simulink model "Automata_Codesys"  (R2018a)
settings: Solver=VariableStepAuto  StartTime=0.0  StopTime=inf  RelTol=1e-3
values from neighbouring files (symbols this model uses):
  bcx = 1000e3    (= 1000000)    [Variables.m]
  bcy = 500e3    (= 500000)    [Variables.m]
  beq1 = 30    [Variables.m]
  beq2 = 18    [Variables.m]
  bw = 30000    [Variables.m]
  g = 9.81    [Variables.m]
  Jeq1 = Jwc+Jmc*(rc^2)    (= 2252)    [Variables.m]
  Jeq2 = Jd+Jmi*(riz^2)    (= 27008)    [Variables.m]
  kcy = 1.3e11    (= 130000000000)    [Variables.m]
  Kw = 1800e3    (= 1800000)    [Variables.m]
  Mc = 50000    [Variables.m]
  Mt = Mc+Jeq1*(1/(Rw^2))    (= 59008)    [Variables.m]
  rc = 15    [Variables.m]
  Rd = 0.75    [Variables.m]
  riz = 30    [Variables.m]
  Rw = 0.5    [Variables.m]
  Y_t0 = 45    [Variables.m]
undefined symbols (not defined in the file or in its folder): AlturaInicialBarco, AlturaInicialMuelle, cont_muelle_masa, contenedores, PObjetivo_fijo, PObjetivo_incremental, x_der, x_izq, Y_inf_barco, Y_max, Y_muelle, Y_sb
libraries: opclib x5
settings Model: Creator=Santiago  LastModifiedBy=Santiago

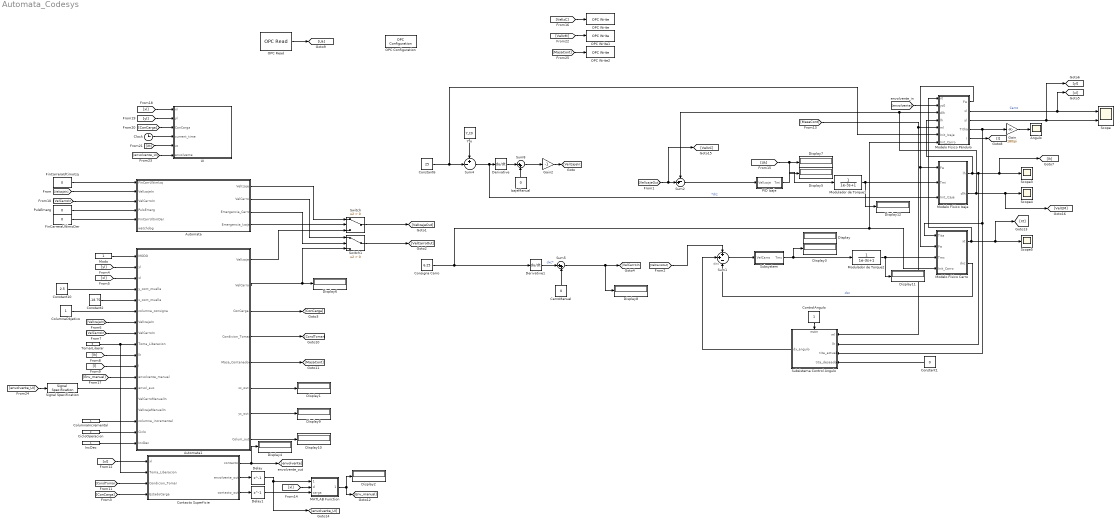
== system Automata_Codesys ==
  note: dxc
  Angulo : Scope
  Automata : Stateflow chart  TreatAsAtomicUnit=on
  Automata1 : Stateflow chart  TreatAsAtomicUnit=on
  CarroManual : Constant  Value=0
  CicloOperacion : Constant  Value=2
  Clock : Clock
  ColumnaIncremental : Constant
  ColumnaObjetivo : Constant
  Consigna Carro : Constant  Value=6.25
  Constant1 : Constant  Value=0
  Constant10 : Constant  Value=2.5
  Constant2 : Constant  Value=-18.75
  Constant6 : Constant  Value=25
  Contacto Superficie : Stateflow chart  TreatAsAtomicUnit=on
  ControlAngulo : Constant
  Delay : Delay  DelayLength=1  InitialCondition=0
  Delay1 : Delay  DelayLength=1  InitialCondition=0
  Derivative : Derivative
  Derivative1 : Derivative
  Display{,1..12} (13 alike) : Display
  FinCarreraUltimoDer : Constant  Value=0
  FinCarreraUltimoIzq : Constant  Value=0
  Gain : Gain  Gain=180/pi
  Gain2 : Gain  Gain=-1
  IncDec : Constant
  IzajeManual : Constant  Value=0
  MATLAB Function : MATLAB Function  TreatAsAtomicUnit=on
  "Modelo Físico Carro " : Subsystem
  Modelo Físico Izaje : Subsystem
  "Modelo Físico Péndulo " : Subsystem
  Modo : Constant
  Modulador de Torque1 : TransferFcn  Denominator=[1e-3 1]
  Modulador de Torque2 : TransferFcn  Denominator=[1e-3 1]
  OPC Configuration : opclib/OPC Configuration  opcServers=localhost/CoDeSys.OPC.DA/100  errMissingItems=Error  errReadWrite=Warn  errShutdown=Error  errRTViolation=Warn  rtEnable=on  speedup=1  showLatency=off  beingUsed=on
      settings: SourceProductName=OPC Toolbox  SourceProductBaseCode=OT
  OPC Read : opclib/OPC Read  serverHost=localhost  serverID=CoDeSys.OPC.DA  itemIDs=Automata.Application.SFC_NIVEL_2.Uk  readMode=Synchronous (cache)  dataType=double  updateRate=1  showQual=off  showTS=off  tsMode=Seconds since start
      settings: SourceProductName=OPC Toolbox  SourceProductBaseCode=OT
  OPC Write : opclib/OPC Write  serverHost=localhost  serverID=CoDeSys.OPC.DA  itemIDs=Automata.Application.SFC_NIVEL_2.VelIzc  writeMode=Synchronous  updateRate=1
      settings: SourceProductName=OPC Toolbox  SourceProductBaseCode=OT
  OPC Write1 : opclib/OPC Write  serverHost=localhost  serverID=CoDeSys.OPC.DA  itemIDs=Automata.Application.SFC_NIVEL_2.VelIzm  writeMode=Synchronous  updateRate=1
      settings: SourceProductName=OPC Toolbox  SourceProductBaseCode=OT
  OPC Write2 : opclib/OPC Write  serverHost=localhost  serverID=CoDeSys.OPC.DA  itemIDs=Automata.Application.SFC_NIVEL_2.Masa_Cont  writeMode=Synchronous  updateRate=1
      settings: SourceProductName=OPC Toolbox  SourceProductBaseCode=OT
  PID Izaje : Subsystem
  PulsEmerg : Constant  Value=0
  Scope : Scope  NumInputPorts=2
  Scope3 : Scope
  Scope4 : Scope
  Scope5 : Scope
  Signal Specification : SignalSpecification  Dimensions=[2,161]
  Subsistema Control Angulo : Subsystem
  Subsystem : Subsystem
  Sum1 : Sum  Inputs=++-
  Sum2 : Sum  Inputs=-+|
  Sum4 : Sum  Inputs=+-|
  Sum5 : Sum  Inputs=|++
  Sum8 : Sum  Inputs=|++
  Switch : Switch  Criteria=u2 > Threshold
  Switch1 : Switch  Criteria=u2 > Threshold
  TomarLiberar : Constant  Value=0
  UI : Stateflow chart  TreatAsAtomicUnit=on  SystemSampleTime=1
  Yto : Constant  Value=Y_t0
  wires:
  Consigna Carro/1 -> "Modelo Físico Carro "/4(Init_Carro), "Modelo Físico Péndulo "/7(Init_Carro), Derivative1/1
  Sum4/1 -> Modelo Físico Izaje/3(Init_Izaje), Derivative/1  "*diz"
  PulsEmerg/1 -> Automata/4(PulsEmerg)
  Automata/1(VelIzaje) -> Switch/1
  Automata/3(Emergencia_Carro) -> Switch1/2
  Automata/2(VelCarro) -> Switch1/1
  [xl] -> Contacto Superficie/1(xl)
  Automata1/3(ConCarga) -> [ConCarga]
  [VelCarroIn] -> Automata/3(VelCarroIn)
  CicloOperacion/1 -> Automata1/17(Ciclo)
  [envolvente_UI] -> Signal Specification/1
  Subsystem/1(Tmc) -> Display3/1, Modulador de Torque2/1
  [yl] -> Automata1/2(yl)
  Automata/4(Emergencia_Izaje) -> Switch/2
  IncDec/1 -> Automata1/18(IncDec)
  Sum8/1 -> Gain2/1
  [CondTomar] -> Contacto Superficie/3(Condicion_Tomar)
  Derivative/1 -> Sum8/1
  [ConCarga] -> Contacto Superficie/4(EstadoCarga)
  Constant2/1 -> Automata1/5(x_cont_muelle)
  [VelCarroOut] -> Sum1/1
  Automata1/4(Condicion_Tomar) -> [CondTomar]
  Automata1/6(xc_out) -> Display1/1
  Yto/1 -> Sum4/1
  [MasaCont] -> Subsistema Control Angulo/1(ml), "Modelo Físico Péndulo "/5(ml)
  [VelIzajeIn] -> Automata/2(VelIzajeIn)
  FinCarreraUltimoDer/1 -> Automata/5(FinCarrUltimDer)
  [ConCarga] -> UI/3(ConCarga)
  Clock/1 -> UI/4(current_time)
  Automata1/7(yc_out) -> Display9/1
  ColumnaIncremental/1 -> Automata1/16(columna_incremental)
  [envolvente_UI] -> UI/6(envolvente)
  Signal Specification/1 -> Automata1/13(envol_aux)
  [Xt] -> UI/5(xt)
  Sum5/1 -> Display8/1, [VelCarroIn]
  ColumnaObjetivo/1 -> Automata1/6(columna_consigna)
  [lh] -> Automata1/10(lh)
  [xl] -> MATLAB Function/2(xl)
  Contacto Superficie/2(envolvente_out) -> Delay/1
  Subsistema Control Angulo/1(dx_angulo) -> Sum1/2
  "Modelo Físico Péndulo "/4(Titha) -> Gain/1, Subsistema Control Angulo/3(tita_actual), "Modelo Físico Carro "/1(Tita)
  Sum2/1 -> PID Izaje/1(VelIzaje)
  MATLAB Function/1(altura_manual) -> Display2/1, [Env_manual]
  Derivative1/1 -> Sum5/1  "dxc*"
  [Env_manual] -> Automata1/12(envolvente_manual)
  Sum1/1 -> Subsystem/1(VelCarro)
  Constant1/1 -> Subsistema Control Angulo/4(tita_deseado)
  Delay/1 -> [envolvente_UI], MATLAB Function/1(envolventes)
  Contacto Superficie/3(contacto_out) -> Delay1/1
  [yl] -> UI/2(yl)
  CarroManual/1 -> Sum5/2
  [xl] -> Automata1/3(xl)
  [VelCarroIn] -> Automata1/8(VelCarroIn)
  Constant10/1 -> Automata1/4(y_cont_muelle)
  [xl] -> UI/1(xl)
  Modo/1 -> Automata1/1(MODO)
  Contacto Superficie/1(contacto) -> Display4/1, [envolvente]
  "Modelo Físico Carro "/2(dxc) -> Sum1/3  "dxc"
  ControlAngulo/1 -> Subsistema Control Angulo/Enable
  Switch1/1 -> [VelCarroOut]
  [VelIzajeIn] -> Automata1/7(VelIzajeIn)
  Automata1/8(Colum_out) -> Display10/1
  "Modelo Físico Carro "/1(xt) -> "Modelo Físico Péndulo "/1(xt), [Xt], Scope5/1
  "Modelo Físico Péndulo "/1(Fw) -> "Modelo Físico Carro "/2(Fw), Modelo Físico Izaje/1(Fw)
  [l] -> Automata1/11(l)
  TomarLiberar/1 -> Contacto Superficie/2(Toma_Liberacion), Automata1/9(Toma_Liberacion)
  Automata1/5(Masa_Contenedor) -> [MasaCont]
  [envolvente] -> "Modelo Físico Péndulo "/2(yc0)
  Constant6/1 -> "Modelo Físico Péndulo "/6(Init_Izaje), Sum4/2
  Gain2/1 -> [VelIzajeIn]
  Modelo Físico Izaje/1(lh) -> Scope3/1, [lh], Subsistema Control Angulo/2(lh), "Modelo Físico Péndulo "/4(lh)
  Delay1/1 -> MATLAB Function/3(carga)
  [VelIzajeOut] -> [VelIzC], Sum2/2
  "Modelo Físico Péndulo "/5(l) -> [l]
  Automata1/2(VelCarro) -> Display6/1, Switch1/3
  Modelo Físico Izaje/2(dlh) -> [VelIzM], Scope4/1, Sum2/1, "Modelo Físico Péndulo "/3(dlh)
  IzajeManual/1 -> Sum8/2
  Switch/1 -> [VelIzajeOut]
  "Modelo Físico Péndulo "/2(xl) -> [xl], Scope/1  "Carro"
  FinCarreraUltimoIzq/1 -> Automata/1(FinCarrUltimIzq)
  Gain/1 -> Angulo/1
  Automata1/1(VelIzaje) -> Switch/3
  Modulador de Torque1/1 -> Display12/1, Modelo Físico Izaje/2(Tmi)
  Modulador de Torque2/1 -> Display11/1, "Modelo Físico Carro "/3(Tmc)
  PID Izaje/1(Tmi) -> Display5/1
  "Modelo Físico Péndulo "/3(yl) -> Scope/2, [yl]
  OPC Read/1 -> [Uk]
  [Uk] -> Modulador de Torque1/1, Display7/1
  [VelIzC] -> OPC Write/1
  [VelIzM] -> OPC Write1/1
  [MasaCont] -> OPC Write2/1

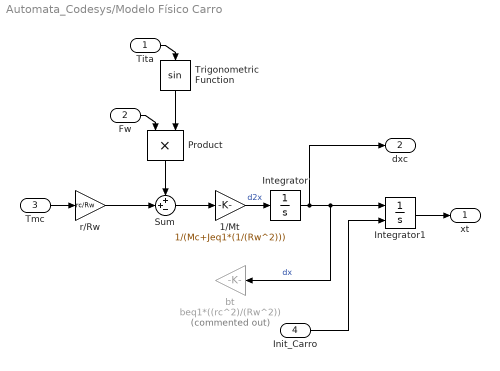
== system Automata_Codesys/Modelo Físico Carro  ==
  Tita : Inport
  Fw : Inport  Port=2
  Tmc : Inport  Port=3
  Init_Carro : Inport  Port=4
  1/Mt : Gain  Gain=1/(Mc+Jeq1*(1/(Rw^2)))
  Integrator : Integrator
  Integrator1 : Integrator  InitialConditionSource=external
  Product : Product
  Sum : Sum  Inputs=++-
  Trigonometric Function : Trigonometry
  bt : Gain  Commented=on  Gain=beq1*((rc^2)/(Rw^2))
  "r/Rw " : Gain  Gain=rc/Rw
  xt : Outport
  dxc : Outport  Port=2
  wires:
  Tita/1 -> Trigonometric Function/1
  Integrator/1 -> dxc/1, bt/1, Integrator1/1  "dx"
  Product/1 -> Sum/1
  "r/Rw "/1 -> Sum/2
  Sum/1 -> 1/Mt/1
  Trigonometric Function/1 -> Product/2
  Integrator1/1 -> xt/1
  1/Mt/1 -> Integrator/1  "d2x"
  Tmc/1 -> "r/Rw "/1
  Fw/1 -> Product/1
  Init_Carro/1 -> Integrator1/2

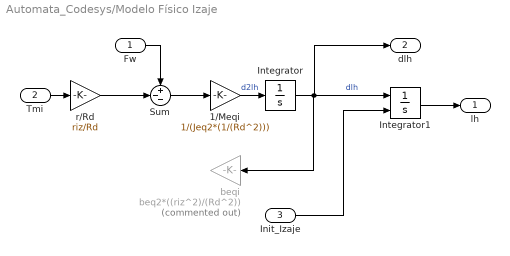
== system Automata_Codesys/Modelo Físico Izaje ==
  Fw : Inport
  Tmi : Inport  Port=2
  Init_Izaje : Inport  Port=3
  1/Meqi : Gain  Gain=1/(Jeq2*(1/(Rd^2)))
  Integrator : Integrator
  Integrator1 : Integrator  InitialConditionSource=external
  Sum : Sum  Inputs=+--
  beqi : Gain  Commented=on  Gain=beq2*((riz^2)/(Rd^2))
  "r/Rd " : Gain  Gain=riz/Rd
  lh : Outport
  dlh : Outport  Port=2
  wires:
  "r/Rd "/1 -> Sum/2
  Sum/1 -> 1/Meqi/1
  Integrator/1 -> beqi/1, dlh/1, Integrator1/1  "dlh"
  Tmi/1 -> "r/Rd "/1
  Integrator1/1 -> lh/1
  1/Meqi/1 -> Integrator/1  "d2lh"
  Fw/1 -> Sum/1
  Init_Izaje/1 -> Integrator1/2

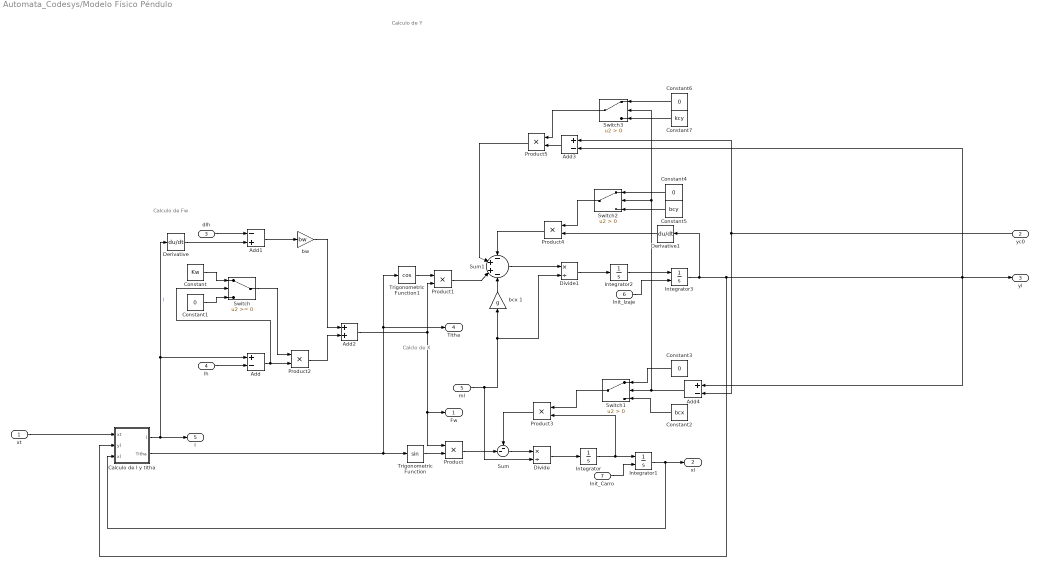
== system Automata_Codesys/Modelo Físico Péndulo  ==
  note: Calculo de Fw
  note: Calclo de X
  note: Calculo de Y
  xt : Inport
  yc0 : Inport  Port=2
  dlh : Inport  Port=3
  lh : Inport  Port=4
  ml : Inport  Port=5
  Init_Izaje : Inport  Port=6
  Init_Carro : Inport  Port=7
  Add : Sum  Inputs=+-
  Add1 : Sum  Inputs=-+
  Add2 : Sum
  Add3 : Sum  Inputs=+-
  Add4 : Sum  Inputs=+-
  Calculo de l y titha : Subsystem
  Constant : Constant  Value=Kw
  Constant{1,3..4,6} (4 alike) : Constant  Value=0
  Constant2 : Constant  Value=bcx
  Constant5 : Constant  Value=bcy
  Constant7 : Constant  Value=kcy
  Derivative : Derivative
  Derivative1 : Derivative
  Divide : Product  Inputs=*/
  Divide1 : Product  Inputs=*/
  Integrator : Integrator
  Integrator1 : Integrator  InitialConditionSource=external
  Integrator2 : Integrator
  Integrator3 : Integrator  InitialConditionSource=external  InitialCondition=20
  Product{,1..5} (6 alike) : Product
  Sum : Sum  Inputs=--|
  Sum1 : Sum  Inputs=-|+|+|-
  Switch : Switch
  Switch1 : Switch  Criteria=u2 > Threshold
  Switch2 : Switch  Criteria=u2 > Threshold
  Switch3 : Switch  Criteria=u2 > Threshold
  Trigonometric Function : Trigonometry
  Trigonometric Function1 : Trigonometry  Operator=cos
  bcx 1 : Gain  Gain=g
  bw : Gain  Gain=bw
  Fw : Outport
  xl : Outport  Port=2
  yl : Outport  Port=3
  Titha : Outport  Port=4
  l : Outport  Port=5
  wires:
  xt/1 -> Calculo de l y titha/1(xt)
  Calculo de l y titha/1(l) -> Add/1, Derivative/1, l/1  "l"
  lh/1 -> Add/2
  Add/1 -> Switch/2, Product2/2
  Add1/1 -> bw/1
  Product2/1 -> Add2/2
  bw/1 -> Add2/1
  dlh/1 -> Add1/1
  Derivative/1 -> Add1/2
  Add2/1 -> Fw/1, Product/1, Product1/2
  Trigonometric Function/1 -> Product/2
  Calculo de l y titha/2(Titha) -> Titha/1, Trigonometric Function1/1, Trigonometric Function/1
  Product/1 -> Sum/2
  Sum/1 -> Divide/1
  Integrator/1 -> Product3/2, Integrator1/1
  Product3/1 -> Sum/1
  Integrator1/1 -> xl/1, Calculo de l y titha/3(xl)
  Trigonometric Function1/1 -> Product1/1
  ml/1 -> Divide1/2, bcx 1/1, Divide/2
  Divide/1 -> Integrator/1
  Product1/1 -> Sum1/3
  bcx 1/1 -> Sum1/4
  yc0/1 -> Add3/1, Add4/2
  Product5/1 -> Sum1/2
  Product4/1 -> Sum1/1
  Integrator2/1 -> Integrator3/1
  Sum1/1 -> Divide1/1
  Divide1/1 -> Integrator2/1
  Switch/1 -> Product2/1
  Constant/1 -> Switch/1
  Constant1/1 -> Switch/3
  Switch1/1 -> Product3/1
  Add4/1 -> Switch1/2, Switch2/2, Switch3/2
  Constant3/1 -> Switch1/1
  Constant2/1 -> Switch1/3
  Switch2/1 -> Product4/1
  Constant4/1 -> Switch2/1
  Constant5/1 -> Switch2/3
  Add3/1 -> Product5/2
  Switch3/1 -> Product5/1
  Constant6/1 -> Switch3/1
  Constant7/1 -> Switch3/3
  Derivative1/1 -> Product4/2
  Init_Carro/1 -> Integrator1/2
  Init_Izaje/1 -> Integrator3/2
  Integrator3/1 -> Add3/2, yl/1, Add4/1, Calculo de l y titha/2(yl), Derivative1/1

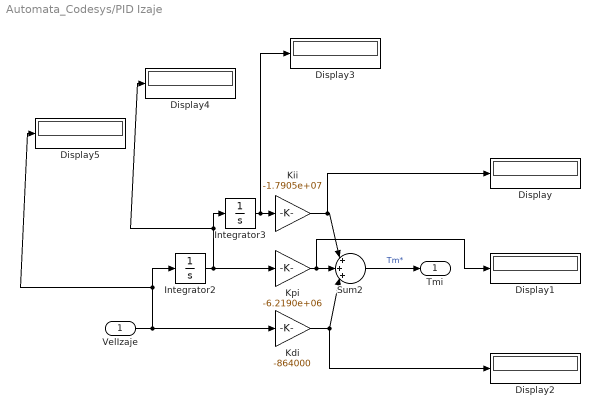
== system Automata_Codesys/PID Izaje ==
  VelIzaje : Inport
  Display{,1..5} (6 alike) : Display
  Integrator2 : Integrator
  Integrator3 : Integrator
  Kdi : Gain  Gain=-864000
  Kii : Gain  Gain=-1.7905e+07
  Kpi : Gain  Gain=-6.2190e+06
  Sum2 : Sum  Inputs=|+++|
  Tmi : Outport
  wires:
  Integrator2/1 -> Display4/1, Integrator3/1, Kpi/1
  Kii/1 -> Display/1, Sum2/1
  VelIzaje/1 -> Kdi/1, Display5/1, Integrator2/1
  Kdi/1 -> Display2/1, Sum2/3
  Sum2/1 -> Tmi/1  "Tm*"
  Kpi/1 -> Display1/1, Sum2/2
  Integrator3/1 -> Display3/1, Kii/1

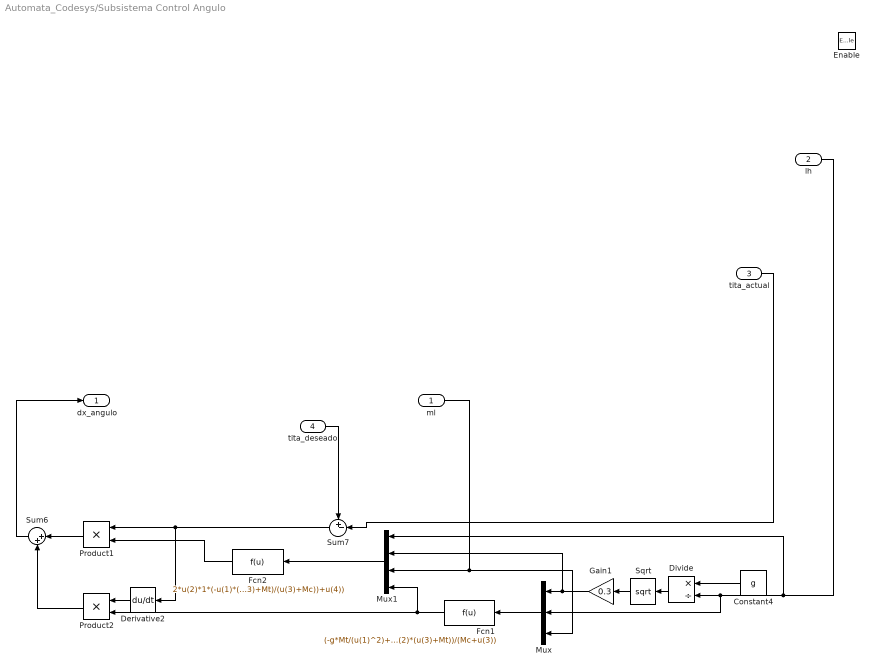
== system Automata_Codesys/Subsistema Control Angulo ==
  ml : Inport
  lh : Inport  Port=2
  tita_actual : Inport  Port=3
  tita_deseado : Inport  Port=4
  Enable : EnablePort
  Constant4 : Constant  Value=g
  Derivative2 : Derivative
  Divide : Product  Inputs=*/
  Fcn1 : Fcn  Expr=(-g*Mt/(u(1)^2)+u(2)*(u(3)+Mt))/(Mc+u(3))
  Fcn2 : Fcn  Expr=2*u(2)*1*(-u(1)*((u(3)+Mt)/(u(3)+Mc))+u(4))
  Gain1 : Gain  Gain=0.3
  Mux : Mux  Inputs=3
  Mux1 : Mux
  Product1 : Product
  Product2 : Product
  Sqrt : Sqrt  SaturateOnIntegerOverflow=on
  Sum6 : Sum  Inputs=|++
  Sum7 : Sum  Inputs=+-|
  dx_angulo : Outport  OutputWhenDisabled=reset  InitialOutput=0
  wires:
  Constant4/1 -> Divide/1
  Fcn1/1 -> Mux1/4, Product2/2
  Mux/1 -> Fcn1/1
  lh/1 -> Mux1/1, Divide/2, Mux/2
  Gain1/1 -> Mux1/2, Mux/1
  Divide/1 -> Sqrt/1
  Derivative2/1 -> Product2/1
  Mux1/1 -> Fcn2/1
  Product1/1 -> Sum6/1
  Fcn2/1 -> Product1/2
  Product2/1 -> Sum6/2
  Sqrt/1 -> Gain1/1
  Sum7/1 -> Product1/1, Derivative2/1
  ml/1 -> Mux/3, Mux1/3
  tita_deseado/1 -> Sum7/1
  tita_actual/1 -> Sum7/2
  Sum6/1 -> dx_angulo/1

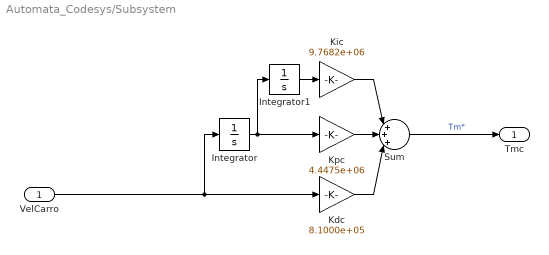
== system Automata_Codesys/Subsystem ==
  VelCarro : Inport
  Integrator : Integrator
  Integrator1 : Integrator
  Kdc : Gain  Gain=8.1000e+05
  Kic : Gain  Gain=9.7682e+06
  Kpc : Gain  Gain=4.4475e+06
  Sum : Sum  Inputs=|+++|
  Tmc : Outport
  wires:
  Integrator1/1 -> Kic/1
  Kic/1 -> Sum/1
  Integrator/1 -> Kpc/1, Integrator1/1
  VelCarro/1 -> Kdc/1, Integrator/1
  Kpc/1 -> Sum/2
  Kdc/1 -> Sum/3
  Sum/1 -> Tmc/1  "Tm*"

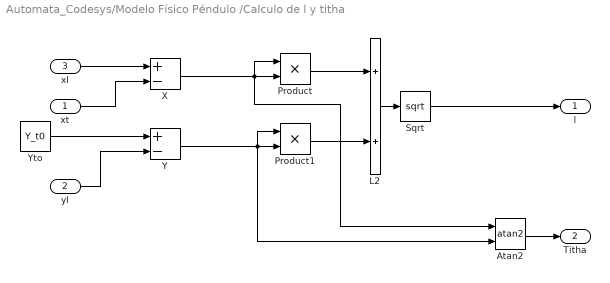
== system Automata_Codesys/Modelo Físico Péndulo /Calculo de l y titha ==
  xt : Inport
  yl : Inport  Port=2
  xl : Inport  Port=3
  Atan2 : Trigonometry  Operator=atan2
  L2 : Sum
  Product : Product
  Product1 : Product
  Sqrt : Sqrt  SaturateOnIntegerOverflow=on
  X : Sum  Inputs=+-
  Y : Sum  Inputs=+-
  Yto : Constant  Value=Y_t0
  l : Outport
  Titha : Outport  Port=2
  wires:
  Y/1 -> Atan2/2, Product1/1, Product1/2
  X/1 -> Product/2, Atan2/1, Product/1
  Product1/1 -> L2/2
  L2/1 -> Sqrt/1
  yl/1 -> Y/2
  Product/1 -> L2/1
  Yto/1 -> Y/1
  xl/1 -> X/1
  Sqrt/1 -> l/1
  xt/1 -> X/2
  Atan2/1 -> Titha/1

== stateflow chart Automata_Codesys/Automata ==
  state NIVEL_0
  state PulsadorEmergencia
    VelIzaje=0;
    VelCarro=0;
    Emergencia_Carro=1;
    Emergencia_Izaje=1;
  state Watchdog
  state SuperVelocidad
    VelIzaje=0;
    VelCarro=VelCarroIn*0.1;
    Emergencia_Carro=-1;
    Emergencia_Izaje=1;
  state FinDeCarreraUltimo
    VelIzaje=VelIzajeIn*0.1;
    VelCarro=0;
    Emergencia_Carro=1;
    Emergencia_Izaje=-1;
  (default) -> NIVEL_0
  NIVEL_0 -> SuperVelocidad [order 3] : [VelIzajeIn>4]
  NIVEL_0 -> PulsadorEmergencia [order 1] : [PulsEmerg==1]
  NIVEL_0 -> FinDeCarreraUltimo [order 2] : [FinCarrUltimDer==1 || FinCarrUltimIzq==1]
  (junction 65) -> NIVEL_0
  NIVEL_0 -> Watchdog [order 4] : [watchdog==1]
  Watchdog -> (junction 65) : [watchdog==0]
  FinDeCarreraUltimo -> (junction 65) : [FinCarrUltimDer==0 && FinCarrUltimIzq==0]
  PulsadorEmergencia -> (junction 65) : [PulsEmerg==0]
  SuperVelocidad -> (junction 65) : [VelIzajeIn<4]
  data: FinCarrUltimIzq input; VelIzajeIn input; VelCarroIn input; PulsEmerg input; FinCarrUltimDer input; VelIzaje output; VelCarro output; Emergencia_Carro output; Emergencia_Izaje output; watchdog input; x_izq parameter; x_der parameter

== stateflow chart Automata_Codesys/Automata1 ==
  state NIVEL_1
    contenedores;
    cont_muelle_masa;
    entry: ConCarga=-1;
    entry: Condicion_Tomar=0;
    entry: Masa_Contenedor=15000;
    entry: pesado=0;
    entry: offset=0;
    note: -Comando operador
        | -Limites normales de oepracion
        | 	-Activacion/desactivacion de control de angulo
        | 	-Fines de carrera
        | 	-Control de Velocidad
        | 	-Estado de carga
        | 		-4 Sensores
        | 		-Twistlook
        | 	-Deteccion cable de izaje flojo
        | 	-Sensor de angulo
    state MODOS [parallel]
      settings: executionOrder=2
      state MANUAL
        state Toma
          if lh>l
          VelIzaje=-0.01;
          else
          VelIzaje=0;
          end
          if Toma_Liberacion==1
          Condicion_Tomar=1;
          ConCarga=1;
          pesado=0;
          end
        state Liberacion
          if lh>l
          VelIzaje=-0.01;
          else
          VelIzaje=0;
          end
          if Toma_Liberacion==-1
          Condicion_Tomar=-1;
          ConCarga=-1;
          pesado=0;
          end
        state Aproximacion
          Condicion_Tomar=0;
          VelCarro=VelCarroIn*0.5;
          VelIzaje=VelIzajeIn*0.5;
          if pesado==1
          offset=2.5;
          elseif pesado==0
          offset=0;
          end
        state Pesaje
          Condicion_Tomar=0;
          if yl<yc+3 && ~(columna_incremental==1 && Ciclo==2)
          VelIzaje=-0.1;
          else
          pesado=1;
          end
        state Movimiento
          VelCarro=VelCarroIn;
          VelIzaje=VelIzajeIn;
        state ProteccionAutomatico
          state FinCarrera
          state FinCarreraDerecho
            state VelCarro
              VelCarro=VelCarroIn;
              VelIzaje=VelIzajeIn;
            state VelCarroBloqueado
              VelCarro=0;
              VelIzaje=VelIzajeIn;
            (default) -> NIVEL_1.MODOS.MANUAL.ProteccionAutomatico.FinCarreraDerecho.VelCarro
            NIVEL_1.MODOS.MANUAL.ProteccionAutomatico.FinCarreraDerecho.VelCarroBloqueado -> NIVEL_1.MODOS.MANUAL.ProteccionAutomatico.FinCarreraDerecho.VelCarro : [VelCarroIn<0]
            NIVEL_1.MODOS.MANUAL.ProteccionAutomatico.FinCarreraDerecho.VelCarro -> NIVEL_1.MODOS.MANUAL.ProteccionAutomatico.FinCarreraDerecho.VelCarroBloqueado : [VelCarroIn>0]
          state FinCarreraIzquierdo
            state VelCarro
              VelCarro=VelCarroIn;
              VelIzaje=VelIzajeIn;
            state VelCarroBloqueado
              VelCarro=0;
              VelIzaje=VelIzajeIn;
            (default) -> NIVEL_1.MODOS.MANUAL.ProteccionAutomatico.FinCarreraIzquierdo.VelCarro
            NIVEL_1.MODOS.MANUAL.ProteccionAutomatico.FinCarreraIzquierdo.VelCarroBloqueado -> NIVEL_1.MODOS.MANUAL.ProteccionAutomatico.FinCarreraIzquierdo.VelCarro : [VelCarroIn>0]
            NIVEL_1.MODOS.MANUAL.ProteccionAutomatico.FinCarreraIzquierdo.VelCarro -> NIVEL_1.MODOS.MANUAL.ProteccionAutomatico.FinCarreraIzquierdo.VelCarroBloqueado : [VelCarroIn<0]
          (default) -> FinCarrera
          FinCarrera -> FinCarreraDerecho [order 2] : [xl>x_der-5]
          FinCarrera -> FinCarreraIzquierdo [order 1] : [xl<x_izq+5]
        (junction 70) -> Toma [order 1] : [ConCarga==-1]
        (junction 70) -> Liberacion [order 2] : [ConCarga==1]
        Aproximacion -> (junction 70) [order 1] : [(yl==yc+offset && xl<xc+0.1 && xl>xc-0.1) ||(yl==y_cont_muelle+offset && xl<x_cont_muelle+0.1 && xl>x_cont_muelle-0.1)]
        Toma -> Pesaje : [ConCarga==1]
        Liberacion -> Aproximacion : [ConCarga==-1]
        Pesaje -> Aproximacion : [ConCarga==1 && pesado==1]
        Aproximacion -> ProteccionAutomatico [order 3] : [xl>x_der-1 || xl<x_izq+1]
        ProteccionAutomatico -> Aproximacion [order 2] : [xl<x_der-1 && xl>x_izq+1]
        Movimiento -> Aproximacion [order 1] : [(yl<yc+2.5 && xl<xc+1 && xl>xc-1) || (yl<y_cont_muelle+2.5 && xl<x_cont_muelle+1 && xl>x_cont_muelle-1)]
        Aproximacion -> Movimiento [order 2] : [(yl>yc+2.5 && xl>xc+1 && xl<xc-1)||(yl>y_cont_muelle+2.5 && xl>x_cont_muelle+1 && xl<x_cont_muelle-1)]
        (default) -> Movimiento
        Movimiento -> ProteccionAutomatico [order 2] : [xl>x_der-1 || xl<x_izq+1]
        ProteccionAutomatico -> Movimiento [order 1] : [xl<x_der-1 && xl>x_izq+1]
      state AUTOMATICO
        state CONFIGURACION
          x_izq;
          x_der;
          PObjetivo_incremental;
          PObjetivo_fijo;
          Y_inf_barco;
          Y_muelle;
          Y_t0;
          Y_max;
          Y_sb;
          AlturaInicialMuelle;
          AlturaInicialBarco;
        state CICLOS
          VelIzaje=VelIzajeIn;
          VelCarro=VelCarroIn;
          note: -Toma de carga (M) OK
              | -Izaje y traslacion (A)
              | -Parada y descenso (A)
              | -Aproximacion fina (M) OK
              | -Liberacion de carga (M) OK
              | -Retorno vacio (A)
        (default) -> CONFIGURACION
        CONFIGURACION -> CICLOS
      (default) -> MANUAL
      MANUAL -> AUTOMATICO : [MODO==-1 && yl>envolvente_manual && yl>=y_cont_muelle+2.5]
      AUTOMATICO -> MANUAL : [MODO==1 || yl<=envolvente_manual || yl<y_cont_muelle+2.5]
    state CoordenadaConsigna [parallel]
      Colum_out=cont_colum;
      xc=(((columna_consigna+cont_colum)*2.5)-1.25)+5;
      xc_out=xc;
      yc=envol_aux(2,round((30+xc)/0.5)+1);
      yc_out=yc;
      settings: executionOrder=1
    state Masa [parallel]
      settings: executionOrder=4
      state MasaSpreader
        Masa_Contenedor=15000;
      state MasaContenedorMuelle
        Masa_Contenedor=cont_muelle_masa+15000;
      state MasaContenedorBarco
        Masa_Contenedor=contenedores(((yc+20)/2.5), (1+(xc-1.25-5)/2.5))+15000;
      (default) -> MasaSpreader
      (junction 167) -> MasaSpreader : [Condicion_Tomar==-1]
      MasaSpreader -> (junction 169) : [Condicion_Tomar==1]
      MasaContenedorMuelle -> (junction 167)
      (junction 169) -> MasaContenedorMuelle [order 1] : [xl<0]
      MasaContenedorBarco -> (junction 167)
      (junction 169) -> MasaContenedorBarco [order 2] : [xl>4]
    state VelocidadTrayectoria [parallel]
      VelMaxIzaje=((9/4)-((3*sqrt(31/5))/(4)))+(97500/(5000*(sqrt(155)-8)+Masa_Contenedor));
      VelMaxCarro=260000/65000;
      settings: executionOrder=3
      VelocidadTrayectoria -> VelocidadTrayectoria
    state ContenedorIncremental [parallel]
      settings: executionOrder=5
      state NoIncremental
        cont_colum=0;
      state SiIncremental
        state SinActualizar
        state Descarga
          state Decremento
            if (columna_consigna + cont_colum)>1
            cont_colum=cont_colum-1;
            end
          state Esperar
          state Incremento
            if (columna_consigna + cont_colum)<18
            cont_colum=cont_colum+1;
            end
          NIVEL_1.ContenedorIncremental.SiIncremental.Descarga.Esperar -> NIVEL_1.ContenedorIncremental.SiIncremental.Descarga.Decremento [order 1] : [IncDec==-1 && Condicion_Tomar==1]
          NIVEL_1.ContenedorIncremental.SiIncremental.Descarga.Decremento -> NIVEL_1.ContenedorIncremental.SiIncremental.Descarga.Esperar : [Condicion_Tomar==0]
          (default) -> NIVEL_1.ContenedorIncremental.SiIncremental.Descarga.Esperar
          NIVEL_1.ContenedorIncremental.SiIncremental.Descarga.Incremento -> NIVEL_1.ContenedorIncremental.SiIncremental.Descarga.Esperar : [Condicion_Tomar==0]
          NIVEL_1.ContenedorIncremental.SiIncremental.Descarga.Esperar -> NIVEL_1.ContenedorIncremental.SiIncremental.Descarga.Incremento [order 2] : [IncDec==1 && Condicion_Tomar==1]
        state Carga
          state Decremento
            if (columna_consigna + cont_colum)>1
            cont_colum=cont_colum-1;
            end
          state Esperar
          state Incremento
            if (columna_consigna + cont_colum)<18
            cont_colum=cont_colum+1;
            end
          NIVEL_1.ContenedorIncremental.SiIncremental.Carga.Decremento -> NIVEL_1.ContenedorIncremental.SiIncremental.Carga.Esperar : [Condicion_Tomar==0]
          NIVEL_1.ContenedorIncremental.SiIncremental.Carga.Esperar -> NIVEL_1.ContenedorIncremental.SiIncremental.Carga.Decremento [order 1] : [IncDec==-1 && Condicion_Tomar==-1]
          (default) -> NIVEL_1.ContenedorIncremental.SiIncremental.Carga.Esperar
          NIVEL_1.ContenedorIncremental.SiIncremental.Carga.Incremento -> NIVEL_1.ContenedorIncremental.SiIncremental.Carga.Esperar : [Condicion_Tomar==0]
          NIVEL_1.ContenedorIncremental.SiIncremental.Carga.Esperar -> NIVEL_1.ContenedorIncremental.SiIncremental.Carga.Incremento [order 2] : [IncDec==1 && Condicion_Tomar==-1]
        (default) -> SinActualizar
        SinActualizar -> Descarga [order 2] : [Ciclo==2]
        SinActualizar -> Carga [order 1] : [Ciclo==1]
        Carga -> Descarga : [Ciclo==2]
        Descarga -> Carga : [Ciclo==1]
      (default) -> NoIncremental
      NoIncremental -> SiIncremental : [columna_incremental==1]
      SiIncremental -> NoIncremental : [columna_incremental==0]
  (default) -> NIVEL_1
  data: VelIzaje output; VelCarro output; MODO input; yl input; Y_inf_barco parameter; AlturaInicialBarco parameter; AlturaInicialMuelle parameter; PObjetivo_fijo parameter; PObjetivo_incremental parameter; x_izq parameter; x_der parameter; Y_muelle parameter; Y_t0 parameter; Y_max parameter; Y_sb parameter; xl input; y_cont_muelle input; x_cont_muelle input; columna_consigna input; VelIzajeIn input; VelCarroIn input; Toma_Liberacion input; lh input; l input; cont_muelle_masa parameter; contenedores parameter; ConCarga output; Condicion_Tomar output; Masa_Contenedor output; envolvente_manual input; envol_aux input; VelCarroManualIn input; VelIzajeManualIn input; envolvente_contacto local; yc local; xc local; columna_incremental input; cont_colum local =0; xc_out output; yc_out output; Colum_out output; pesado local; offset local; VelMaxIzaje local; VelMaxCarro local; Ciclo input; IncDec input

== stateflow chart Automata_Codesys/Contacto Superficie ==
  state ModeloContacto
    envolvente;
    entry: envolventes=envolvente;
    during: envolvente_out=envolventes;
    state ContactoConstante [parallel]
      settings: executionOrder=2
      state SinContenedor
        contacto=envolventes(2,round((30+xl)/0.5)+1);
        contacto_out=-1;
      state ConContenedor
        contacto=envolventes(2,round((30+xl)/0.5)+1)+2.5;
        contacto_out=1;
      (default) -> SinContenedor
      ConContenedor -> SinContenedor : [EstadoCarga==-1]
      SinContenedor -> ConContenedor : [EstadoCarga==1]
    state ContactoActualizacion [parallel]
      settings: executionOrder=1
      state ContactoNormal
      state ContactoTomar
        index=round((30+xl)/0.5)+1;
        if envolventes(1,index)<=xl
        for i=1:5
        envolventes(2,index-3+i)=envolventes(2,index-3+i)-2.5;
        end
        elseif envolventes(1,index)>xl
        for i=1:5
        envolventes(2,index-4+i)=envolventes(2,index-4+i)-2.5;
        end
        end
      state ContactoLiberar
        index=round((30+xl)/0.5)+1;
        if envolventes(1,index)<=xl
        for i=1:5
        envolventes(2,index-3+i)=envolventes(2,index-3+i)+2.5;
        end
        elseif envolventes(1,index)>xl
        for i=1:5
        envolventes(2,index-4+i)=envolventes(2,index-4+i)+2.5;
        end
        end
      (default) -> ContactoNormal
      ContactoLiberar -> ContactoNormal : [Condicion_Tomar==0]
      ContactoNormal -> ContactoLiberar [order 2] : [Toma_Liberacion==-1 && Condicion_Tomar==1]
      ContactoTomar -> ContactoNormal : [Condicion_Tomar==0]
      ContactoNormal -> ContactoTomar [order 1] : [Toma_Liberacion==1 && Condicion_Tomar==1]
  data: envolvente parameter; xl input; contacto output; envolventes local; Toma_Liberacion input; i local; index local; Condicion_Tomar input; envolvente_out output; yc local; xc local; EstadoCarga input; contacto_out output

== matlab function Automata_Codesys/MATLAB Function ==
  data: envolventes input; altura_manual output; xl input; carga input
function altura_manual = env(envolventes,xl,carga)
altura_manual=zeros(1,1);
envolvente_manual=zeros(2,161);

x=envolventes(1,:);
y=envolventes(2,:);
xnuevo=x;
ynuevo=y;
for i=1:61
    ynuevo(i)=ynuevo(i)+2.5;
end

for i=71:5:length(x)
    if i==71
        if ((y(i-1)-y(i))>2.5 || (y(i+5)-y(i))>2.5)
            aux=max(y(i-1),y(i+5));
            for j=0:4
                ynuevo(i+j)=aux;
            end
        end
        
    else
        
        if i~=length(x) && (y(i-5)-y(i)>2.5 || y(i+5)-y(i)>2.5)
            aux=max(y(i-5),y(i+5));
            for j=0:4
                ynuevo(i+j)=aux;
            end
        else
            if i~=length(x)
                for j=0:4
                    ynuevo(i+j)=y(i);
                end
            else
                ynuevo(i)=y(i);
            end
        end
    end
end
for i=71:length(xnuevo)
    ynuevo(i)=ynuevo(i)+2.5;
end
envolvente_manual(1,:)=xnuevo;
envolvente_manual(2,:)=ynuevo;
if carga==1
    altura_manual=envolvente_manual(2,round((30+xl)/0.5)+1)+2.5;
elseif carga==-1
    altura_manual=envolvente_manual(2,round((30+xl)/0.5)+1);
end
end

== stateflow chart Automata_Codesys/UI ==
  state Graficador
    en: coder.extrinsic('Automatas_Codesys', 'actualizarPosiciones');
    app = Automatas_Codesys();
    during: actualizarPosiciones(app, xl,yl,ConCarga,current_time,xt,envolvente)
  (default) -> Graficador
  data: xl input; yl input; ConCarga input; app local; current_time input; xt input; envolvente input
